simulink model "es4"  (R2022b)
settings: Solver=VariableStepAuto  StartTime=0.0  StopTime=4.8  RelTol=1e-3
settings Model: Creator=adlercohen  LastModifiedBy=adlercohen

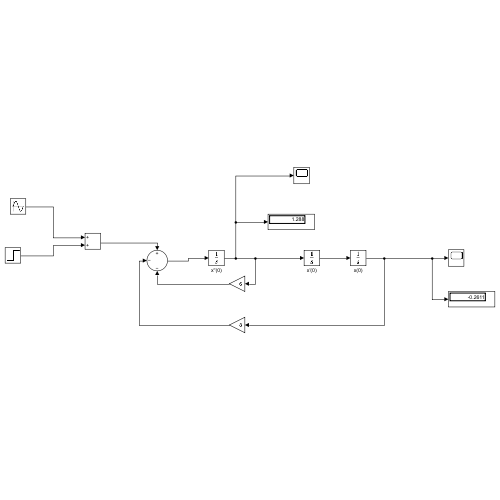
[thumbnail: Simulink's stored preview of the top-level diagram]
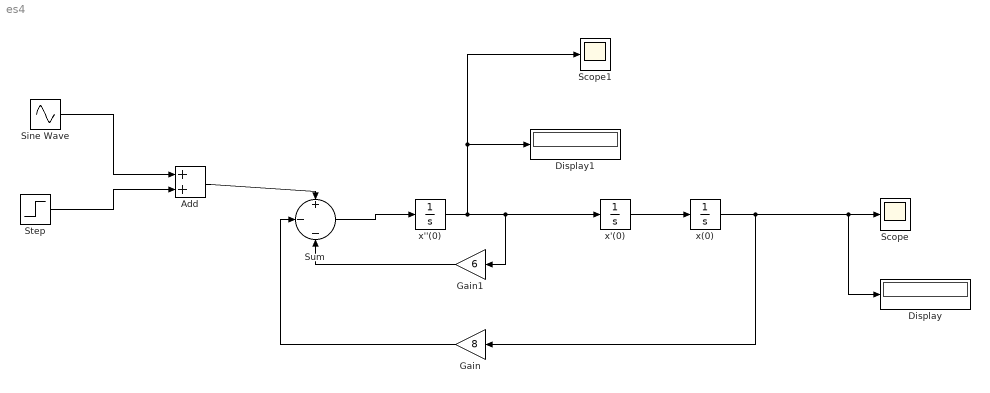
== system es4 ==
  Add : Sum
  Display : Display
  Display1 : Display
  Gain : Gain  Gain=8
  Gain1 : Gain  Gain=6
  Scope : Scope
  Scope1 : Scope
  Sine Wave : Sin  Amplitude=2  Frequency=pi/4  SampleTime=0
  Step : Step  Time=0  After=10  SampleTime=0
  Sum : Sum  Inputs=+|-|-
  x''(0) : Integrator  InitialCondition=1.8
  x'(0) : Integrator
  x(0) : Integrator
  wires:
  x''(0)/1 -> Display1/1, Scope1/1, Gain1/1, x'(0)/1
  Sum/1 -> x''(0)/1
  Gain1/1 -> Sum/3
  Sine Wave/1 -> Add/1
  Gain/1 -> Sum/2
  x'(0)/1 -> x(0)/1
  x(0)/1 -> Scope/1, Display/1, Gain/1
  Step/1 -> Add/2
  Add/1 -> Sum/1
